simulink model "ar_algorithm"  (R2018a)
settings: Solver=VariableStepAuto  StartTime=0.0  StopTime=6  RelTol=1e-3  EnableMultiTasking=on
InitFcn:
  | ar_init
values from neighbouring files (symbols this model uses):
  JL = 2.25    [ar_init.m]    (also in bode_analysis.m)
  Jm = 0.015    [ar_init.m]    (also in bode_analysis.m)
  kf = 0.1    [ar_init.m]    (also in bode_analysis.m)
  Ks = 65    [ar_init.m]    (also in bode_analysis.m)
undefined symbols (not defined in the file or in its folder): DiscIntNeverNeededParam
libraries: dsparch4 x4, simulink x1
settings Model: Creator=LG-PC  LastModifiedBy=LG-PC
settings DataIOCC: LimitDataPoints=on
settings OptimizationCC: LifeSpan=inf
settings DebuggingCC: AllowSymbolicDim=off  LibraryContextMissingDiagnostic=warning  SFUnexpectedBacktrackingDiag=warning  SFNoUnconditionalDefaultTransitionDiag=warning  SFExecutionAtInitializationDiag=none
settings ModelReferenceCC: PropagateSignalLabelsOutOfModel=off
settings CodeAppCC: StateflowObjectComments=on
settings GRTTargetCC: TargetLangStandard=C89/C90 (ANSI)
settings ConfigComp: CovMetricSettings=dw  CovHtmlReporting=on  CovSaveCumulativeToWorkspaceVar=on  CovSaveSingleToWorkspaceVar=on  CovExternalEMLEnable=off

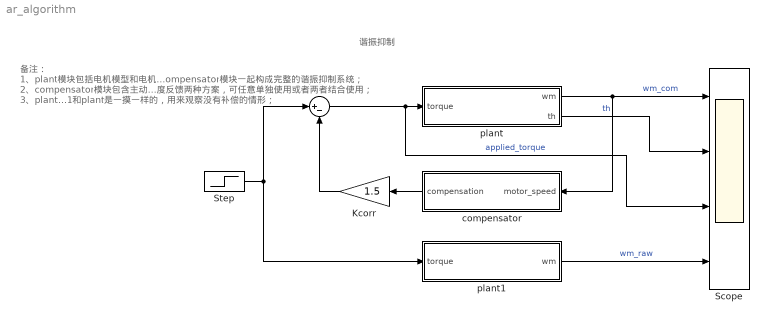
== system ar_algorithm ==
  note: 谐振抑制
  note: 备注：
      | 1、plant模块包括电机模型和电机-负载二质量模型，与compensator模块一起构成完整的谐振抑制系统；
      |
      | 2、compensator模块包含主动阻尼和加速度反馈两种方案，可任意单独使用或者两者结合使用；
      |
      | 3、plant1和plant是一摸一样的，用来观察没有补偿的情形；
  Kcorr : Gain  Gain=1.5
  Scope : Scope  NumInputPorts=4
  Step : Step  After=80  SampleTime=0
  Sum : Sum  Inputs=|+-
  "compensator " : Subsystem
  plant : Subsystem
  plant1 : Subsystem
  wires:
  Sum/1 -> Scope/3, plant/1(torque)  "applied_torque"
  "compensator "/1(compensation) -> Kcorr/1
  Step/1 -> plant1/1(torque), Sum/1
  Kcorr/1 -> Sum/2
  plant/1(wm) -> "compensator "/1(motor_speed), Scope/1  "wm_com"
  plant/2(th) -> Scope/2  "th"
  plant1/1(wm) -> Scope/4  "wm_raw"

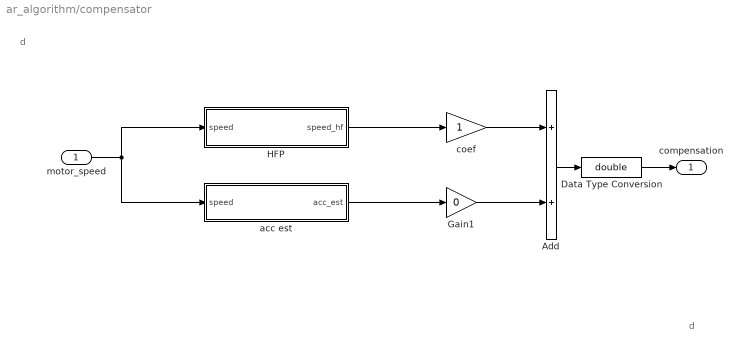
== system ar_algorithm/compensator  ==
  note: d
  note: d
  motor_speed : Inport
  Add : Sum
  Data Type Conversion : DataTypeConversion  OutDataTypeStr=double
  Gain1 : Gain  Gain=0
  HFP : Subsystem
  acc est : Subsystem
  coef : Gain
  compensation : Outport
  wires:
  HFP/1(speed_hf) -> coef/1
  motor_speed/1 -> acc est/1(speed), HFP/1(speed)
  Add/1 -> Data Type Conversion/1
  Gain1/1 -> Add/2
  Data Type Conversion/1 -> compensation/1
  acc est/1(acc_est) -> Gain1/1
  coef/1 -> Add/1

== system ar_algorithm/plant ==
  note: 备注：
      | 1、motor模块用来模拟电机产生转矩的功能，用来生成转矩；
      |
      | 2、mech sys模块包含电机和负载的运动模型，以及两者通过柔性连接所构成的所谓‘二质量模型’；
      |
      | 3、模型的刚度系数和阻尼系数、电机和负载的惯量仅用于展示效果，用于实际问题需要根据具体情况进行修改；
  torque : Inport
  mech sys : Subsystem
  motor : Subsystem
  wm : Outport
  th : Outport  Port=2
  wires:
  mech sys/1(wm) -> motor/1(wm), wm/1
  motor/1(Tm) -> mech sys/1(Te)
  torque/1 -> motor/2(Tc)
  motor/2(Th) -> th/1

== system ar_algorithm/plant1 ==
  note: 备注：
      | 1、motor模块用来模拟电机产生转矩的功能，用来生成转矩；
      |
      | 2、mech sys模块包含电机和负载的运动模型，以及两者通过柔性连接所构成的所谓‘二质量模型’；
      |
      | 3、模型的刚度系数和阻尼系数、电机和负载的惯量仅用于展示效果，用于实际问题需要根据具体情况进行修改；
  torque : Inport
  mech sys : Subsystem
  motor : Subsystem
  wm : Outport
  wires:
  torque/1 -> motor/2(Tc)
  motor/1(Tm) -> mech sys/1(Te)
  mech sys/1(wm) -> motor/1(wm), wm/1

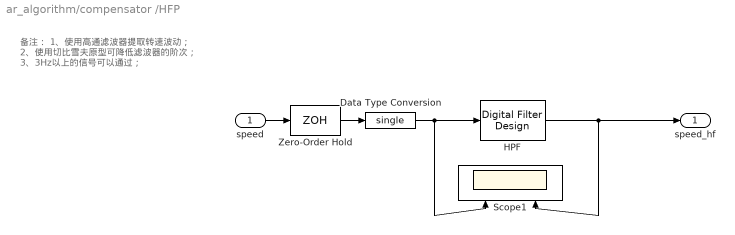
== system ar_algorithm/compensator /HFP ==
  note: 备注：
      | 1、使用高通滤波器提取转速波动；
      |
      | 2、使用切比雪夫原型可降低滤波器的阶次；
      |
      | 3、3Hz以上的信号可以通过；
  speed : Inport
  Data Type Conversion : DataTypeConversion  OutDataTypeStr=single
  "HPF " : dsparch4/Digital Filter Design  mwdsp_browser_bugfix_var=off
  Scope1 : Scope  NumInputPorts=2
  Zero-Order Hold : ZeroOrderHold  SampleTime=1/1000
  speed_hf : Outport
  wires:
  speed/1 -> Zero-Order Hold/1
  Zero-Order Hold/1 -> Data Type Conversion/1
  Data Type Conversion/1 -> "HPF "/1, Scope1/1
  "HPF "/1 -> speed_hf/1, Scope1/2

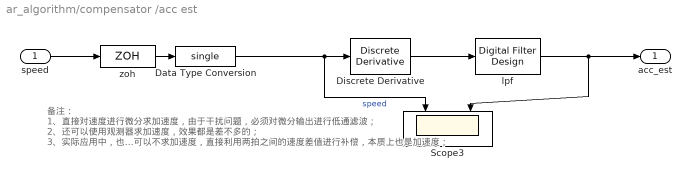
== system ar_algorithm/compensator /acc est ==
  note: 备注：
      | 1、直接对速度进行微分求加速度，由于干扰问题，必须对微分输出进行低通滤波；
      | 2、还可以使用观测器求加速度，效果都是差不多的；
      | 3、实际应用中，也可以不求加速度，直接利用两拍之间的速度差值进行补偿，本质上也是加速度；
  speed : Inport
  Data Type Conversion : DataTypeConversion  OutDataTypeStr=single
  Discrete Derivative : simulink/Discrete/Discrete Derivative  gainval=1.0  ICPrevScaledInput=0.0  OutMin=[]  OutMax=[]  OutDataType=fixdt(1, 16)  OutScaling=2^-10  DoSatur=off
  Scope3 : Scope  NumInputPorts=2
  lpf : dsparch4/Digital Filter Design  mwdsp_browser_bugfix_var=off
  zoh : ZeroOrderHold  SampleTime=1/1000
  acc_est : Outport
  wires:
  speed/1 -> zoh/1
  zoh/1 -> Data Type Conversion/1
  Data Type Conversion/1 -> Scope3/1, Discrete Derivative/1  "speed"
  lpf/1 -> acc_est/1, Scope3/2
  Discrete Derivative/1 -> lpf/1

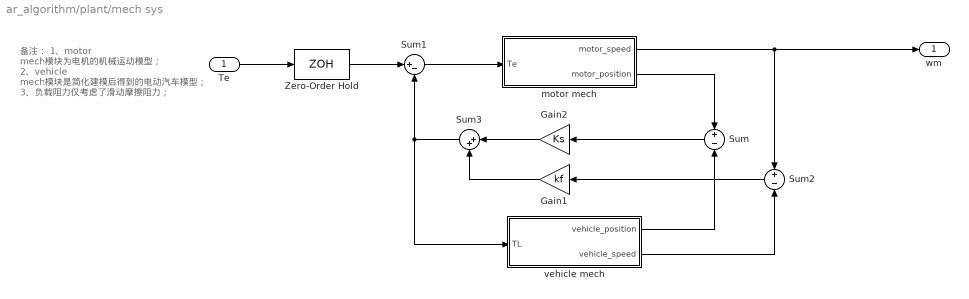
== system ar_algorithm/plant/mech sys ==
  note: 备注：
      | 1、motor mech模块为电机的机械运动模型；
      | 2、vehicle mech模块是简化建模后得到的电动汽车模型；
      |
      | 3、负载阻力仅考虑了滑动摩擦阻力；
  Te : Inport
  Gain1 : Gain  Gain=kf
  Gain2 : Gain  Gain=Ks
  Sum : Sum  Inputs=+|-
  Sum1 : Sum  Inputs=|+-
  Sum2 : Sum  Inputs=+|-
  Sum3 : Sum  Inputs=|++
  Zero-Order Hold : ZeroOrderHold  SampleTime=1/10000
  motor mech : Subsystem
  vehicle mech : Subsystem
  wm : Outport
  wires:
  Te/1 -> Zero-Order Hold/1
  Gain2/1 -> Sum3/1
  Sum/1 -> Gain2/1
  Sum1/1 -> motor mech/1(Te)
  motor mech/2(motor_position) -> Sum/1
  vehicle mech/1(vehicle_position) -> Sum/2
  vehicle mech/2(vehicle_speed) -> Sum2/2
  Sum2/1 -> Gain1/1
  Gain1/1 -> Sum3/2
  Sum3/1 -> Sum1/2, vehicle mech/1(TL)
  motor mech/1(motor_speed) -> wm/1, Sum2/1
  Zero-Order Hold/1 -> Sum1/1

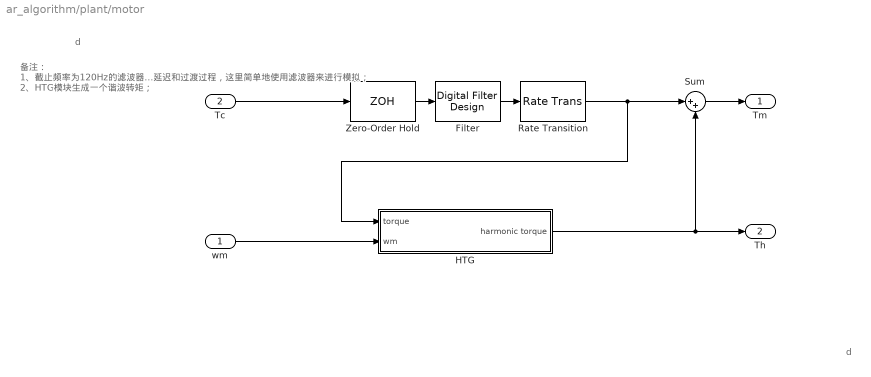
== system ar_algorithm/plant/motor ==
  note: 备注：
      | 1、截止频率为120Hz的滤波器用来模拟电机转矩的延迟。对于实际电机，在实际输出转矩和转矩指令之间一定存在延迟和过渡过程，这里简单地使用滤波器来进行模拟；
      | 2、HTG模块生成一个谐波转矩；
  note: d
  note: d
  wm : Inport
  Tc : Inport  Port=2
  Filter : dsparch4/Digital Filter Design  mwdsp_browser_bugfix_var=off
  HTG : Subsystem
  Rate Transition : RateTransition
  Sum : Sum  Inputs=|++
  Zero-Order Hold : ZeroOrderHold  SampleTime=1/1000
  Tm : Outport
  Th : Outport  Port=2
  wires:
  Tc/1 -> Zero-Order Hold/1
  Sum/1 -> Tm/1
  Rate Transition/1 -> HTG/1(torque), Sum/1
  wm/1 -> HTG/2(wm)
  HTG/1(harmonic torque) -> Sum/2, Th/1
  Zero-Order Hold/1 -> Filter/1
  Filter/1 -> Rate Transition/1

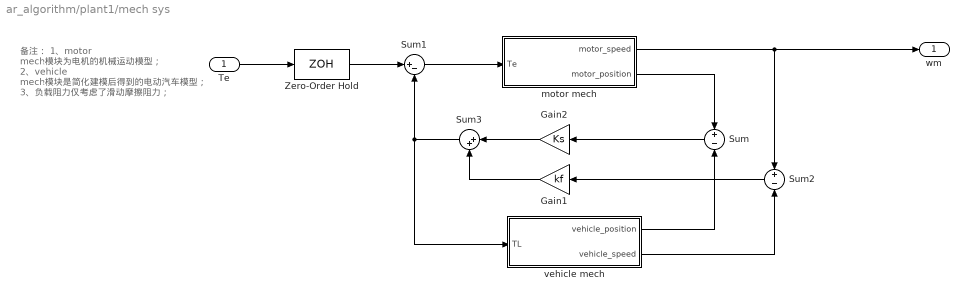
== system ar_algorithm/plant1/mech sys ==
  note: 备注：
      | 1、motor mech模块为电机的机械运动模型；
      | 2、vehicle mech模块是简化建模后得到的电动汽车模型；
      |
      | 3、负载阻力仅考虑了滑动摩擦阻力；
  Te : Inport
  Gain1 : Gain  Gain=kf
  Gain2 : Gain  Gain=Ks
  Sum : Sum  Inputs=+|-
  Sum1 : Sum  Inputs=|+-
  Sum2 : Sum  Inputs=+|-
  Sum3 : Sum  Inputs=|++
  Zero-Order Hold : ZeroOrderHold  SampleTime=1/10000
  motor mech : Subsystem
  vehicle mech : Subsystem
  wm : Outport
  wires:
  Zero-Order Hold/1 -> Sum1/1
  motor mech/1(motor_speed) -> Sum2/1, wm/1
  Sum3/1 -> vehicle mech/1(TL), Sum1/2
  Gain1/1 -> Sum3/2
  Sum2/1 -> Gain1/1
  vehicle mech/2(vehicle_speed) -> Sum2/2
  vehicle mech/1(vehicle_position) -> Sum/2
  motor mech/2(motor_position) -> Sum/1
  Sum1/1 -> motor mech/1(Te)
  Sum/1 -> Gain2/1
  Gain2/1 -> Sum3/1
  Te/1 -> Zero-Order Hold/1

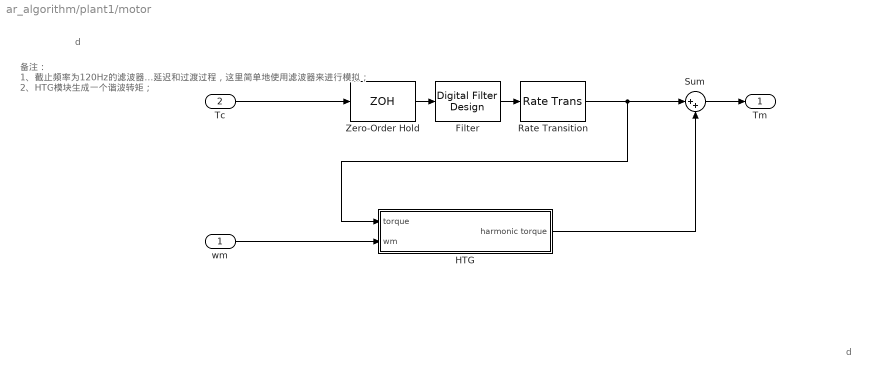
== system ar_algorithm/plant1/motor ==
  note: d
  note: d
  note: 备注：
      | 1、截止频率为120Hz的滤波器用来模拟电机转矩的延迟。对于实际电机，在实际输出转矩和转矩指令之间一定存在延迟和过渡过程，这里简单地使用滤波器来进行模拟；
      | 2、HTG模块生成一个谐波转矩；
  wm : Inport
  Tc : Inport  Port=2
  Filter : dsparch4/Digital Filter Design  mwdsp_browser_bugfix_var=off
  HTG : Subsystem
  Rate Transition : RateTransition
  Sum : Sum  Inputs=|++
  Zero-Order Hold : ZeroOrderHold  SampleTime=1/1000
  Tm : Outport
  wires:
  Filter/1 -> Rate Transition/1
  Zero-Order Hold/1 -> Filter/1
  HTG/1(harmonic torque) -> Sum/2
  wm/1 -> HTG/2(wm)
  Rate Transition/1 -> Sum/1, HTG/1(torque)
  Sum/1 -> Tm/1
  Tc/1 -> Zero-Order Hold/1

== system ar_algorithm/plant/mech sys/motor mech ==
  note: d
  note: d
  Te : Inport
  Discrete-Time Integrator : DiscreteIntegrator  SampleTime=-1  ICPrevOutput=DiscIntNeverNeededParam  ICPrevScaledInput=DiscIntNeverNeededParam
  Discrete-Time Integrator1 : DiscreteIntegrator  SampleTime=-1  ICPrevOutput=DiscIntNeverNeededParam  ICPrevScaledInput=DiscIntNeverNeededParam
  motor_Inertia : Gain  Gain=1/Jm
  motor_speed : Outport
  motor_position : Outport  Port=2
  wires:
  Discrete-Time Integrator/1 -> Discrete-Time Integrator1/1, motor_speed/1
  motor_Inertia/1 -> Discrete-Time Integrator/1
  Te/1 -> motor_Inertia/1
  Discrete-Time Integrator1/1 -> motor_position/1

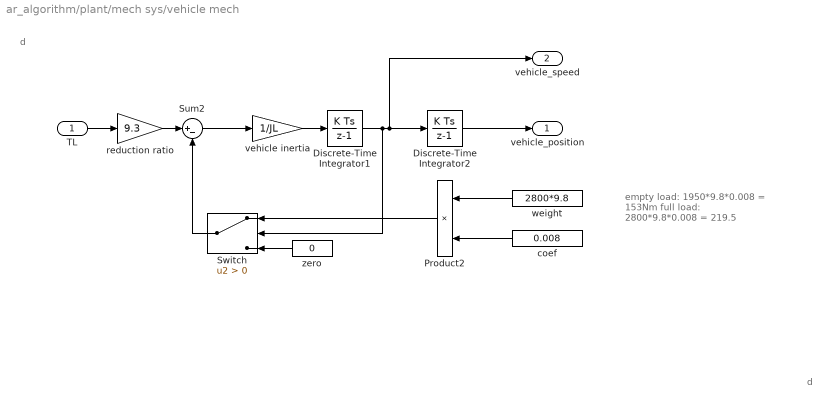
== system ar_algorithm/plant/mech sys/vehicle mech ==
  note: empty load:
      | 1950*9.8*0.008 = 153Nm
      | full load:
      | 2800*9.8*0.008 = 219.5
  note: d
  note: d
  TL : Inport
  Discrete-Time Integrator1 : DiscreteIntegrator  SampleTime=-1  ICPrevOutput=DiscIntNeverNeededParam  ICPrevScaledInput=DiscIntNeverNeededParam
  Discrete-Time Integrator2 : DiscreteIntegrator  SampleTime=-1  ICPrevOutput=DiscIntNeverNeededParam  ICPrevScaledInput=DiscIntNeverNeededParam
  Product2 : Product
  Sum2 : Sum  Inputs=|+-
  Switch : Switch  Criteria=u2 > Threshold
  coef : Constant  Value=0.008
  "reduction ratio " : Gain  Gain=9.3
  vehicle inertia : Gain  Gain=1/JL
  weight : Constant  Value=2800*9.8
  zero : Constant  Value=0
  vehicle_position : Outport
  vehicle_speed : Outport  Port=2
  wires:
  Discrete-Time Integrator2/1 -> vehicle_position/1
  Sum2/1 -> vehicle inertia/1
  TL/1 -> "reduction ratio "/1
  vehicle inertia/1 -> Discrete-Time Integrator1/1
  Switch/1 -> Sum2/2
  coef/1 -> Product2/2
  Product2/1 -> Switch/1
  weight/1 -> Product2/1
  zero/1 -> Switch/3
  "reduction ratio "/1 -> Sum2/1
  Discrete-Time Integrator1/1 -> Switch/2, Discrete-Time Integrator2/1, vehicle_speed/1

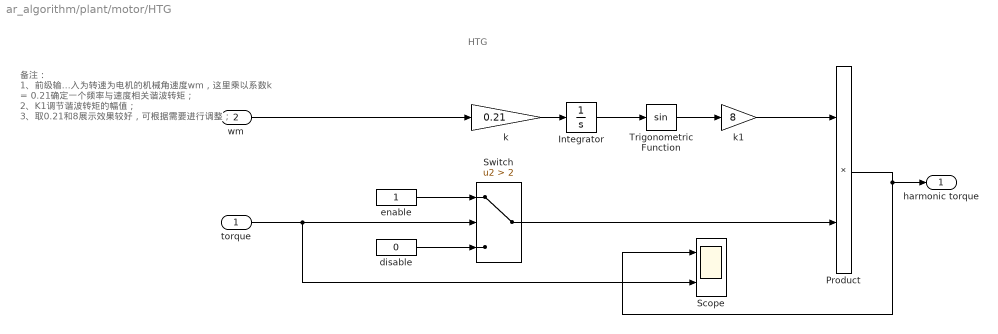
== system ar_algorithm/plant/motor/HTG ==
  note: HTG
  note: 备注：
      | 1、前级输入为转速为电机的机械角速度wm，这里乘以系数k = 0.21确定一个频率与速度相关谐波转矩；
      |
      | 2、K1调节谐波转矩的幅值；
      |
      | 3、取0.21和8展示效果较好，可根据需要进行调整；
  torque : Inport
  wm : Inport  Port=2
  Integrator : Integrator
  Product : Product
  Scope : Scope  NumInputPorts=2
  Switch : Switch  Criteria=u2 > Threshold  Threshold=2
  Trigonometric Function : Trigonometry
  disable : Constant  Value=0
  enable : Constant
  k : Gain  Gain=0.21
  k1 : Gain  Gain=8
  harmonic torque : Outport
  wires:
  Trigonometric Function/1 -> k1/1
  Integrator/1 -> Trigonometric Function/1
  k/1 -> Integrator/1
  enable/1 -> Switch/1
  torque/1 -> Scope/2, Switch/2
  disable/1 -> Switch/3
  k1/1 -> Product/1
  Product/1 -> Scope/1, harmonic torque/1
  Switch/1 -> Product/2
  wm/1 -> k/1

== system ar_algorithm/plant1/mech sys/motor mech ==
  note: d
  note: d
  Te : Inport
  Discrete-Time Integrator : DiscreteIntegrator  SampleTime=-1  ICPrevOutput=DiscIntNeverNeededParam  ICPrevScaledInput=DiscIntNeverNeededParam
  Discrete-Time Integrator1 : DiscreteIntegrator  SampleTime=-1  ICPrevOutput=DiscIntNeverNeededParam  ICPrevScaledInput=DiscIntNeverNeededParam
  motor_Inertia : Gain  Gain=1/Jm
  motor_speed : Outport
  motor_position : Outport  Port=2
  wires:
  Discrete-Time Integrator1/1 -> motor_position/1
  Te/1 -> motor_Inertia/1
  motor_Inertia/1 -> Discrete-Time Integrator/1
  Discrete-Time Integrator/1 -> motor_speed/1, Discrete-Time Integrator1/1

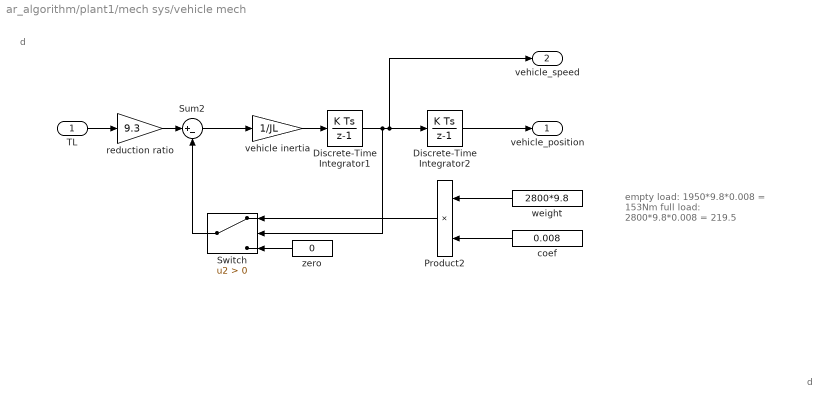
== system ar_algorithm/plant1/mech sys/vehicle mech ==
  note: d
  note: d
  note: empty load:
      | 1950*9.8*0.008 = 153Nm
      | full load:
      | 2800*9.8*0.008 = 219.5
  TL : Inport
  Discrete-Time Integrator1 : DiscreteIntegrator  SampleTime=-1  ICPrevOutput=DiscIntNeverNeededParam  ICPrevScaledInput=DiscIntNeverNeededParam
  Discrete-Time Integrator2 : DiscreteIntegrator  SampleTime=-1  ICPrevOutput=DiscIntNeverNeededParam  ICPrevScaledInput=DiscIntNeverNeededParam
  Product2 : Product
  Sum2 : Sum  Inputs=|+-
  Switch : Switch  Criteria=u2 > Threshold
  coef : Constant  Value=0.008
  "reduction ratio " : Gain  Gain=9.3
  vehicle inertia : Gain  Gain=1/JL
  weight : Constant  Value=2800*9.8
  zero : Constant  Value=0
  vehicle_position : Outport
  vehicle_speed : Outport  Port=2
  wires:
  Discrete-Time Integrator1/1 -> vehicle_speed/1, Discrete-Time Integrator2/1, Switch/2
  "reduction ratio "/1 -> Sum2/1
  zero/1 -> Switch/3
  weight/1 -> Product2/1
  Product2/1 -> Switch/1
  coef/1 -> Product2/2
  Switch/1 -> Sum2/2
  vehicle inertia/1 -> Discrete-Time Integrator1/1
  TL/1 -> "reduction ratio "/1
  Sum2/1 -> vehicle inertia/1
  Discrete-Time Integrator2/1 -> vehicle_position/1

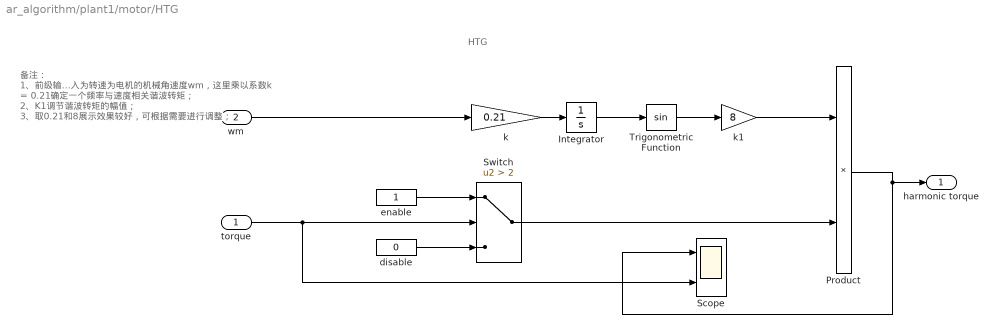
== system ar_algorithm/plant1/motor/HTG ==
  note: 备注：
      | 1、前级输入为转速为电机的机械角速度wm，这里乘以系数k = 0.21确定一个频率与速度相关谐波转矩；
      |
      | 2、K1调节谐波转矩的幅值；
      |
      | 3、取0.21和8展示效果较好，可根据需要进行调整；
  note: HTG
  torque : Inport
  wm : Inport  Port=2
  Integrator : Integrator
  Product : Product
  Scope : Scope  NumInputPorts=2
  Switch : Switch  Criteria=u2 > Threshold  Threshold=2
  Trigonometric Function : Trigonometry
  disable : Constant  Value=0
  enable : Constant
  k : Gain  Gain=0.21
  k1 : Gain  Gain=8
  harmonic torque : Outport
  wires:
  wm/1 -> k/1
  Switch/1 -> Product/2
  Product/1 -> harmonic torque/1, Scope/1
  k1/1 -> Product/1
  disable/1 -> Switch/3
  torque/1 -> Switch/2, Scope/2
  enable/1 -> Switch/1
  k/1 -> Integrator/1
  Integrator/1 -> Trigonometric Function/1
  Trigonometric Function/1 -> k1/1
